simulink model "TractionControl"  (R2020a)
settings: Solver=FixedStepAuto  StartTime=0.0  StopTime=10.0  FixedStep=0.001  RelTol=1e-3  EnableMultiTasking=on
settings Model: Creator=Harjot  LastModifiedBy=Harjot
settings OptimizationCC: LifeSpan=inf
settings DebuggingCC: SFUnexpectedBacktrackingDiag=warning  SFNoUnconditionalDefaultTransitionDiag=warning  ArithmeticOperatorsInVariantConditions=warning
settings SFSimCC: SimUseLocalCustomCode=off  CustomCodeUndefinedFunction=UseInterfaceOnly
settings RTWCC: RTWUseLocalCustomCode=off
settings CodeAppCC: StateflowObjectComments=on
settings GRTTargetCC: TargetLangStandard=C89/C90 (ANSI)
settings ConfigComp: CovMetricSettings=dw  CovHtmlReporting=on  CovSaveCumulativeToWorkspaceVar=on  CovSaveSingleToWorkspaceVar=on  CovExternalEMLEnable=off

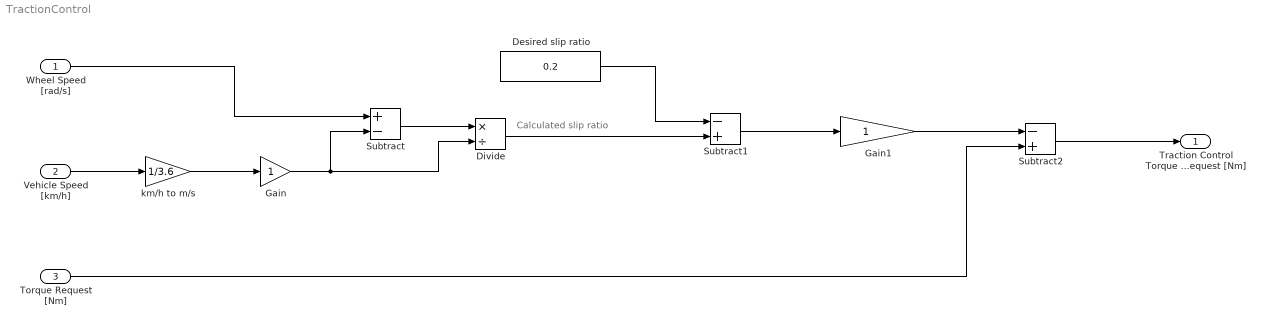
== system TractionControl ==
  note: Calculated slip ratio
  Wheel Speed [rad/s] : Inport
  Vehicle Speed [km/h] : Inport  Port=2
  Torque Request [Nm] : Inport  Port=3
  Desired slip ratio : Constant  Value=0.2
  Divide : Product  Inputs=*/
  Gain : Gain
  Gain1 : Gain
  Subtract : Sum  Inputs=+-
  Subtract1 : Sum  Inputs=-+
  Subtract2 : Sum  Inputs=-+
  km/h to m/s : Gain  Gain=1/3.6
  Traction Control Torque Request [Nm] : Outport  VectorParamsAs1DForOutWhenUnconnected=off
  wires:
  Vehicle Speed [km/h]/1 -> km/h to m/s/1
  km/h to m/s/1 -> Gain/1
  Wheel Speed [rad/s]/1 -> Subtract/1
  Gain/1 -> Divide/2, Subtract/2
  Subtract/1 -> Divide/1
  Desired slip ratio/1 -> Subtract1/1
  Divide/1 -> Subtract1/2
  Subtract1/1 -> Gain1/1
  Gain1/1 -> Subtract2/1
  Torque Request [Nm]/1 -> Subtract2/2
  Subtract2/1 -> Traction Control Torque Request [Nm]/1
